simulink model "lateral_calibration"  (R2021b)
settings: Solver=VariableStepAuto  StartTime=0.0  StopTime=50  RelTol=1e-3
libraries: Solver_SF x1
settings Model: Creator=Li Ang  LastModifiedBy=Li Ang

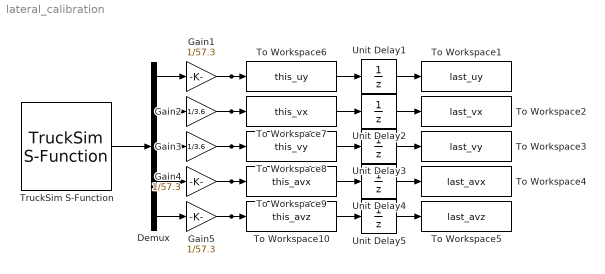
== system lateral_calibration ==
  Demux : Demux  Outputs=5
  Gain1 : Gain  Gain=1/57.3
  Gain2 : Gain  Gain=1/3.6
  Gain3 : Gain  Gain=1/3.6
  Gain4 : Gain  Gain=1/57.3
  Gain5 : Gain  Gain=1/57.3
  To Workspace1 : ToWorkspace  VariableName=last_uy  SaveFormat=Timeseries  SampleTime=0.01
  To Workspace10 : ToWorkspace  VariableName=this_avz  SaveFormat=Timeseries  SampleTime=0.01
  To Workspace2 : ToWorkspace  VariableName=last_vx  SaveFormat=Timeseries  SampleTime=0.01
  To Workspace3 : ToWorkspace  VariableName=last_vy  SaveFormat=Timeseries  SampleTime=0.01
  To Workspace4 : ToWorkspace  VariableName=last_avx  SaveFormat=Timeseries  SampleTime=0.01
  To Workspace5 : ToWorkspace  VariableName=last_avz  SaveFormat=Timeseries  SampleTime=0.01
  To Workspace6 : ToWorkspace  VariableName=this_uy  SaveFormat=Timeseries  SampleTime=0.01
  To Workspace7 : ToWorkspace  VariableName=this_vx  SaveFormat=Timeseries  SampleTime=0.01
  To Workspace8 : ToWorkspace  VariableName=this_vy  SaveFormat=Timeseries  SampleTime=0.01
  To Workspace9 : ToWorkspace  VariableName=this_avx  SaveFormat=Timeseries  SampleTime=0.01
  TruckSim S-Function : Solver_SF/TruckSim S-Function  Priority=1  SIMFILE=simfile.sim  Run_RTs=off  vs_state_ind=Run  StopMode_ind=Vehicle Model
      settings: SourceProductName=TruckSim S-Function
  Unit Delay{1..5} (5 alike) : UnitDelay  SampleTime=-1  HasFrameUpgradeWarning=on
  wires:
  TruckSim S-Function/1 -> Demux/1
  Demux/1 -> Gain1/1
  Demux/2 -> Gain2/1
  Demux/3 -> Gain3/1
  Demux/4 -> Gain4/1
  Demux/5 -> Gain5/1
  Gain1/1 -> Unit Delay1/1, To Workspace6/1
  Gain2/1 -> Unit Delay2/1, To Workspace7/1
  Gain3/1 -> Unit Delay3/1, To Workspace8/1
  Gain4/1 -> Unit Delay4/1, To Workspace9/1
  Gain5/1 -> Unit Delay5/1, To Workspace10/1
  Unit Delay1/1 -> To Workspace1/1
  Unit Delay2/1 -> To Workspace2/1
  Unit Delay3/1 -> To Workspace3/1
  Unit Delay4/1 -> To Workspace4/1
  Unit Delay5/1 -> To Workspace5/1
